simulink model "Simulink_UDP"  (R2020a)
settings: Solver=VariableStepAuto  StartTime=0.0  StopTime=10.0  RelTol=1e-3
libraries: instrumentlib x1
settings Model: EnablePacing=on  Creator=david  LastModifiedBy=david

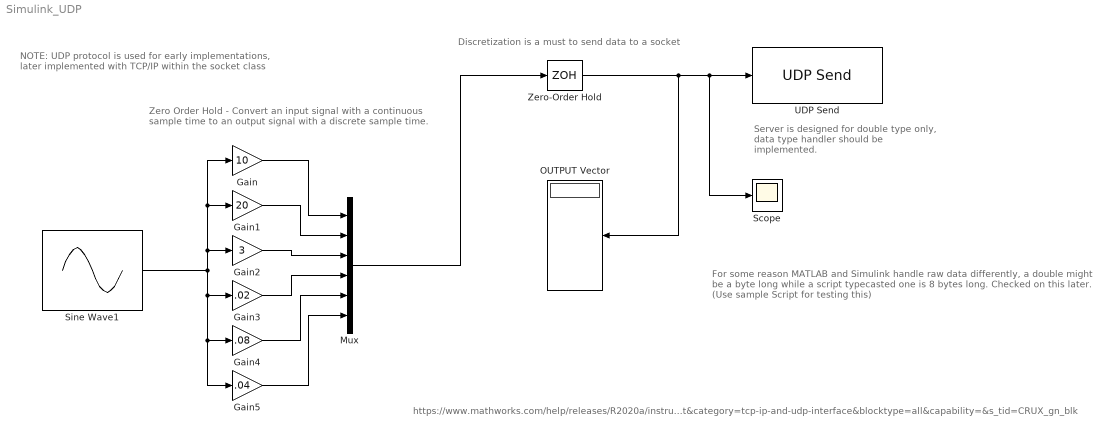
== system Simulink_UDP ==
  note: https://www.mathworks.com/help/releases/R2020a/instrument/referencelist.html?type=block&listtype=cat&category=tcp-ip-and-udp-interface&blocktype=all&capability=&s_tid=CRUX_gn_blk
  note: NOTE: UDP protocol is used for early implementations, later implemented with TCP/IP within the socket class
  note: Zero Order Hold - Convert an input signal with a continuous
      | sample time to an output signal with a discrete sample time.
  note: For some reason MATLAB and Simulink handle raw data differently,
      | a double might be a byte long while a script typecasted one is 8 bytes long.
      | Checked on this later. (Use sample Script for testing this)
  note: Server is designed for double type only, data type handler should be
      | implemented.
  note: Discretization is a must to send data to a socket
  Gain : Gain  Gain=10
  Gain1 : Gain  Gain=20
  Gain2 : Gain  Gain=3
  Gain3 : Gain  Gain=.02
  Gain4 : Gain  Gain=.08
  Gain5 : Gain  Gain=.04
  Mux : Mux  Inputs=6
  OUTPUT Vector : Display
  Scope : Scope
  Sine Wave1 : Sin  SampleTime=0
  UDP Send : instrumentlib/UDP Send  Host=127.0.0.1  Port=50010  LocalPort=-1  EnablePortSharing=off  ByteOrder=LittleEndian  OutputDatagramPacketSize=1024  EnableBlockingMode=on  LocalAddress=0.0.0.0
  Zero-Order Hold : ZeroOrderHold  SampleTime=.01
  wires:
  Sine Wave1/1 -> Gain5/1, Gain4/1, Gain3/1, Gain/1, Gain1/1, Gain2/1
  Gain5/1 -> Mux/6
  Gain1/1 -> Mux/2
  Gain2/1 -> Mux/3
  Mux/1 -> Zero-Order Hold/1
  Gain/1 -> Mux/1
  Gain3/1 -> Mux/4
  Gain4/1 -> Mux/5
  Zero-Order Hold/1 -> OUTPUT Vector/1, Scope/1, UDP Send/1
